simulink model "model_no_linear_mpc"  (R2022a)
settings: Solver=VariableStepAuto  StartTime=0  StopTime=100  RelTol=1e-3
values from neighbouring files (symbols this model uses):
  amplitude_entrada = 1    [ball_and_beam_pfc.m]
  bool_degrau = 1    [ball_and_beam_pfc.m]
  C = [0 0 1 0]    [ball_and_beam_pfc.m]
  g = 9.8    [ball_and_beam_pfc.m]    (also in nonlinear_ball_and_beam.m)
  Jv = (1/2) * mv * L^2    (= 0.058703125)    [ball_and_beam_pfc.m]    (also in nonlinear_ball_and_beam.m)
  L = 0.425    [ball_and_beam_pfc.m]    (also in nonlinear_ball_and_beam.m)
  mb = 0.064    [ball_and_beam_pfc.m]    (also in nonlinear_ball_and_beam.m)
  mv = 0.65    [ball_and_beam_pfc.m]    (also in nonlinear_ball_and_beam.m)
libraries: mpclib x1
settings Model: Creator=Notebook_Artur  LastModifiedBy=Notebook_Artur

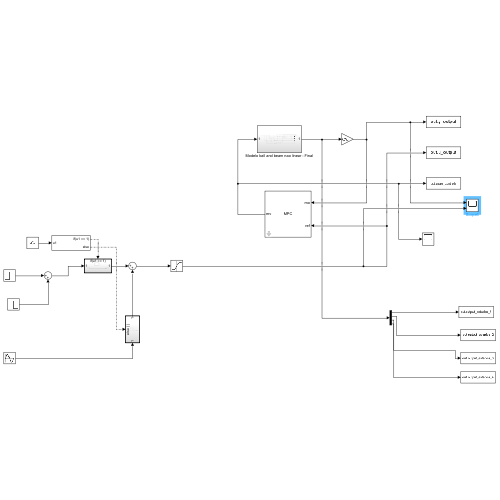
[thumbnail: Simulink's stored preview of the top-level diagram]
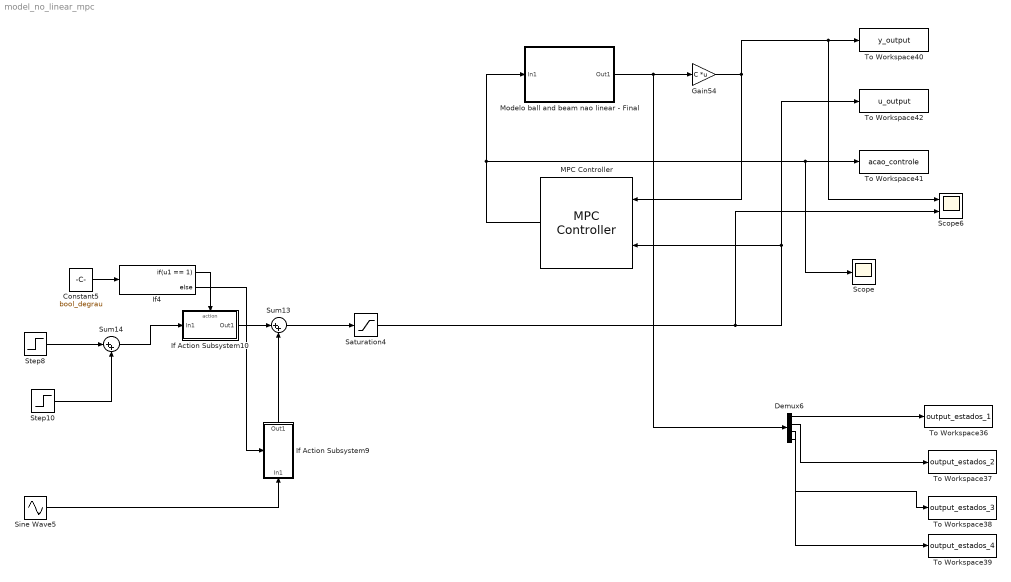
== system model_no_linear_mpc ==
  Constant5 : Constant  Value=bool_degrau
  Demux6 : Demux
  Gain54 : Gain  Gain=C  Multiplication=Matrix(K*u)
  If Action Subsystem10 : Subsystem  TreatAsAtomicUnit=on
  If Action Subsystem9 : Subsystem  TreatAsAtomicUnit=on
  If4 : If  IfExpression=u1 == 1
  MPC Controller : mpclib/MPC Controller  SCDEnableBlockLinearizationSpecification=on  mpcobj=mpc_no_linear  is_multiple=0  enable_value=0  return_u0=off  updateMPCinCallerWorkspace=on  md_inport=off  mv_inport=off  uref_inport=off  return_cost=off  return_mvseq=off  return_qpstatus=off  return_xseq=off  return_state=off  return_ovseq=off  state_inport=off  umin_inport=off  umax_inport=off  ymin_inport=off  ymax_inport=off  cc_inport=off  ywt_inport=off  uwt_inport=off  duwt_inport=off  rhoeps_inport=off  pm_inport=off  MaximumP=10  HorizonChoice=FixedHorizon  n_ts=0.1  n_p=10  n_mv=1  n_md=0  n_ud=0  n_mo=1  n_uo=0  BlockDataType=double  SampleTimeInherited=off  switch_inport=off
  Modelo ball and beam nao linear - Final : Subsystem
  Saturation4 : Saturate  UpperLimit=L/2  LowerLimit=-L/2
  Scope : Scope
  Scope6 : Scope  NumInputPorts=2
  Sine Wave5 : Sin  Amplitude=amplitude_entrada  Frequency=0.1  SampleTime=0
  Step10 : Step  Time=100  After=-2*amplitude_entrada  SampleTime=0
  Step8 : Step  After=amplitude_entrada  SampleTime=0
  Sum13 : Sum  Inputs=|++
  Sum14 : Sum  Inputs=|++
  To Workspace36 : ToWorkspace  VariableName=output_estados_1  SaveFormat=Timeseries  SampleTime=-1
  To Workspace37 : ToWorkspace  VariableName=output_estados_2  SaveFormat=Timeseries  SampleTime=-1
  To Workspace38 : ToWorkspace  VariableName=output_estados_3  SaveFormat=Timeseries  SampleTime=-1
  To Workspace39 : ToWorkspace  VariableName=output_estados_4  SaveFormat=Timeseries  SampleTime=-1
  To Workspace40 : ToWorkspace  VariableName=y_output  SaveFormat=Timeseries  SampleTime=-1
  To Workspace41 : ToWorkspace  VariableName=acao_controle  SaveFormat=Timeseries  SampleTime=-1
  To Workspace42 : ToWorkspace  VariableName=u_output  SaveFormat=Timeseries  SampleTime=-1
  wires:
  Saturation4/1 -> Scope6/2, MPC Controller/2, To Workspace42/1
  Sum13/1 -> Saturation4/1
  If Action Subsystem10/1(Out1) -> Sum13/1
  Step8/1 -> Sum14/1
  Demux6/1 -> To Workspace36/1
  Demux6/2 -> To Workspace37/1
  Modelo ball and beam nao linear - Final/1(Out1) -> Demux6/1, Gain54/1
  Demux6/3 -> To Workspace38/1
  Sum14/1 -> If Action Subsystem10/1(In1)
  Sine Wave5/1 -> If Action Subsystem9/1(In1)
  If Action Subsystem9/1(Out1) -> Sum13/2
  Gain54/1 -> MPC Controller/1, Scope6/1, To Workspace40/1
  Demux6/4 -> To Workspace39/1
  If4/2 -> If Action Subsystem9/Action
  Step10/1 -> Sum14/2
  If4/1 -> If Action Subsystem10/Action
  MPC Controller/1 -> Scope/1, To Workspace41/1, Modelo ball and beam nao linear - Final/1(In1)
  Constant5/1 -> If4/1

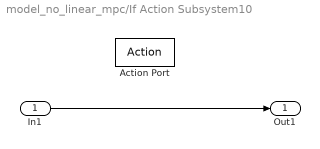
== system model_no_linear_mpc/If Action Subsystem10 ==
  In1 : Inport
  Action Port : ActionPort  ActionPortLabel=if(u1 == 1)
  Out1 : Outport
  wires:
  In1/1 -> Out1/1

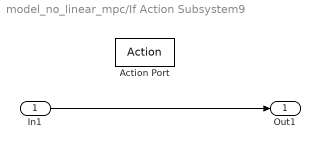
== system model_no_linear_mpc/If Action Subsystem9 ==
  In1 : Inport
  Action Port : ActionPort  ActionPortLabel=else
  Out1 : Outport
  wires:
  In1/1 -> Out1/1

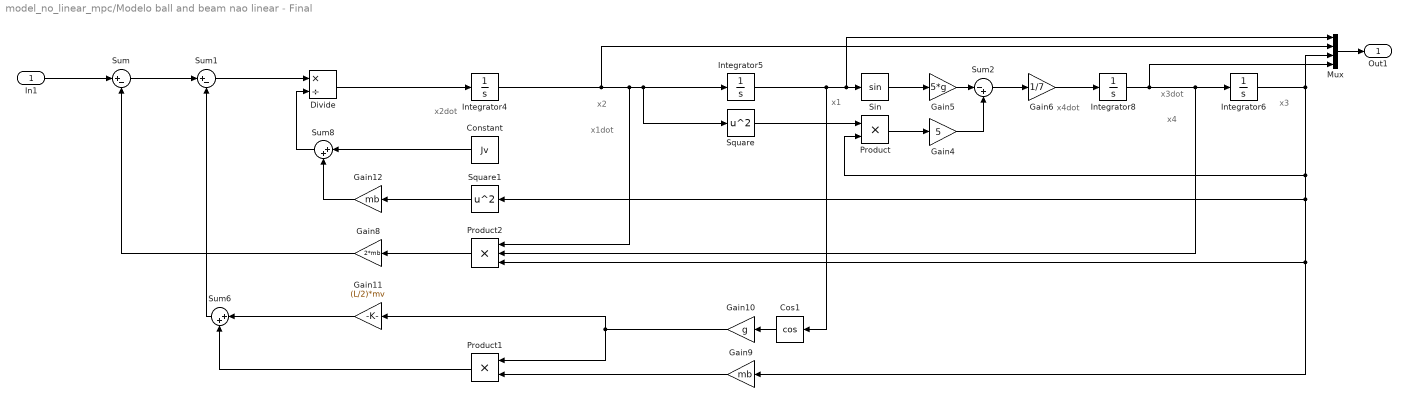
== system model_no_linear_mpc/Modelo ball and beam nao linear - Final ==
  note: x3
  note: x3dot
  note: x4
  note: x4dot
  note: x1
  note: x1dot
  note: x2dot
  note: x2
  In1 : Inport
  Constant : Constant  Value=Jv
  Cos1 : Trigonometry  Operator=cos
  Divide : Product  Inputs=*/
  Gain10 : Gain  Gain=g
  Gain11 : Gain  Gain=(L/2)*mv
  Gain12 : Gain  Gain=mb
  Gain4 : Gain  Gain=5
  Gain5 : Gain  Gain=5*g
  Gain6 : Gain  Gain=1/7
  Gain8 : Gain  Gain=2*mb
  Gain9 : Gain  Gain=mb
  Integrator{4..6,8} (4 alike) : Integrator
  Mux : Mux
  Product : Product
  Product1 : Product
  Product2 : Product  Inputs=3
  Sin : Trigonometry
  Square : Math  Operator=square
  Square1 : Math  Operator=square
  Sum : Sum  Inputs=|+-
  Sum1 : Sum  Inputs=|+-
  Sum2 : Sum  Inputs=|-+
  Sum6 : Sum  Inputs=|++
  Sum8 : Sum  Inputs=|++
  Out1 : Outport
  wires:
  Integrator8/1 -> Mux/4, Product2/2, Integrator6/1
  Integrator5/1 -> Cos1/1, Mux/1, Sin/1
  Sum6/1 -> Sum1/2
  Sum2/1 -> Gain6/1
  Gain10/1 -> Product1/1, Gain11/1
  Square/1 -> Product/1
  Integrator6/1 -> Mux/3, Gain9/1, Product2/3, Square1/1, Product/2
  Gain11/1 -> Sum6/1
  Gain12/1 -> Sum8/2
  Gain6/1 -> Integrator8/1
  Gain4/1 -> Sum2/2
  Gain9/1 -> Product1/2
  Cos1/1 -> Gain10/1
  Divide/1 -> Integrator4/1
  Product2/1 -> Gain8/1
  Product/1 -> Gain4/1
  Square1/1 -> Gain12/1
  Sum8/1 -> Divide/2
  Product1/1 -> Sum6/2
  Constant/1 -> Sum8/1
  Mux/1 -> Out1/1
  Gain5/1 -> Sum2/1
  Sin/1 -> Gain5/1
  Gain8/1 -> Sum/2
  Sum1/1 -> Divide/1
  Sum/1 -> Sum1/1
  Integrator4/1 -> Mux/2, Product2/1, Square/1, Integrator5/1
  In1/1 -> Sum/1
